simulink model "thermal_project"  (R2021a)
settings: Solver=FixedStepDiscrete  StartTime=0.0  StopTime=10.0  FixedStep=0.1  RelTol=1e-3
libraries: simulink x3
settings Model: Creator=vayne  LastModifiedBy=vayne
settings OptimizationCC: DefaultParameterBehavior=Inlined  EnhancedBackFolding=on  PassReuseOutputArgsAs=Individual arguments  ZeroExternalMemoryAtStartup=off  ZeroInternalMemoryAtStartup=off  OptimizeBlockOrder=speed  DifferentSizesBufferReuse=on  OptimizationCustomize=off  EfficientTunableParamExpr=on
settings DebuggingCC: ParameterTunabilityLossMsg=error
settings HardwareCC: ProdBitPerPointer=32  ProdBitPerSizeT=32  ProdBitPerPtrDiffT=32  ProdLargestAtomicInteger=Long  ProdLargestAtomicFloat=Double  ProdWordSize=32  ProdHWDeviceType=ARM Compatible->ARM Cortex-M
settings SFSimCC: MATLABDynamicMemAlloc=off
settings RTWCC: Description=Create Visual C/C++ Solution File for Embedded Coder  SystemTargetFile=ert.tlc  GenCodeOnly=on  TemplateMakefile=ert_default_tmf  Toolchain=MinGW64 | gmake (64-bit Windows)
settings CodeAppCC: ForceParamTrailComments=on  IgnoreCustomStorageClasses=off  OperatorAnnotations=on  SimulinkDataObjDesc=on  SFDataObjDesc=on  InsertBlockDesc=on
settings ERTTargetCC: TargetLangStandard=C99 (ISO)  GenerateSampleERTMain=on  InlinedParameterPlacement=NonHierarchical  ERTCustomFileTemplate=example_file_process.tlc

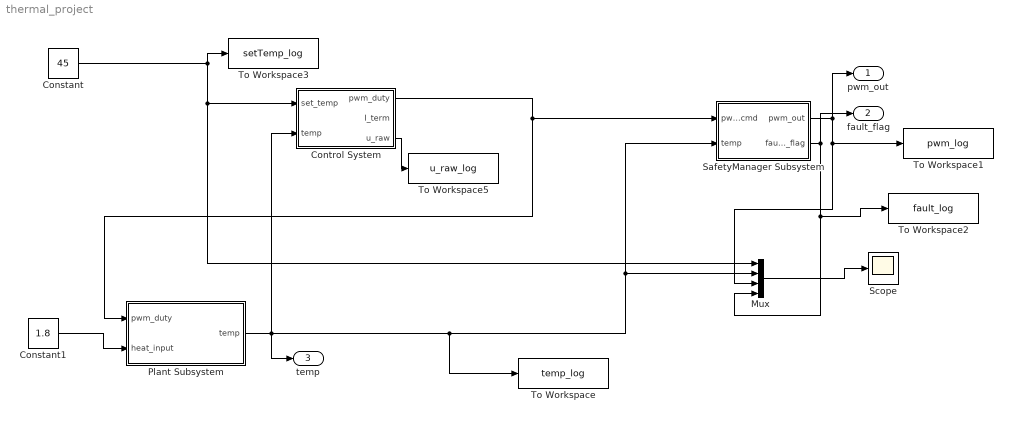
== system thermal_project ==
  Constant : Constant  Value=45
  Constant1 : Constant  Value=1.8
  Control System : Subsystem
  Mux : Mux
  Plant Subsystem : Subsystem
  SafetyManager Subsystem : Subsystem
  Scope : Scope
  To Workspace : ToWorkspace  VariableName=temp_log  SaveFormat=Structure With Time  SampleTime=-1
  To Workspace1 : ToWorkspace  VariableName=pwm_log  SaveFormat=Structure With Time  SampleTime=-1
  To Workspace2 : ToWorkspace  VariableName=fault_log  SaveFormat=Structure With Time  SampleTime=-1
  To Workspace3 : ToWorkspace  VariableName=setTemp_log  SaveFormat=Structure With Time  SampleTime=-1
  To Workspace5 : ToWorkspace  VariableName=u_raw_log  SaveFormat=Structure With Time  SampleTime=-1
  pwm_out : Outport
  fault_flag : Outport  Port=2
  temp : Outport  Port=3
  wires:
  Constant/1 -> Mux/1, Control System/1(set_temp), To Workspace3/1
  Control System/3(u_raw) -> To Workspace5/1
  SafetyManager Subsystem/2(fault_flag) -> To Workspace2/1, Mux/4, fault_flag/1
  Plant Subsystem/1(temp) -> temp/1, Control System/2(temp), To Workspace/1, Mux/2, SafetyManager Subsystem/2(temp)
  Mux/1 -> Scope/1
  SafetyManager Subsystem/1(pwm_out) -> To Workspace1/1, Mux/3, pwm_out/1
  Control System/1(pwm_duty) -> SafetyManager Subsystem/1(pwm_cmd), Plant Subsystem/1(pwm_duty)
  Constant1/1 -> Plant Subsystem/2(heat_input)

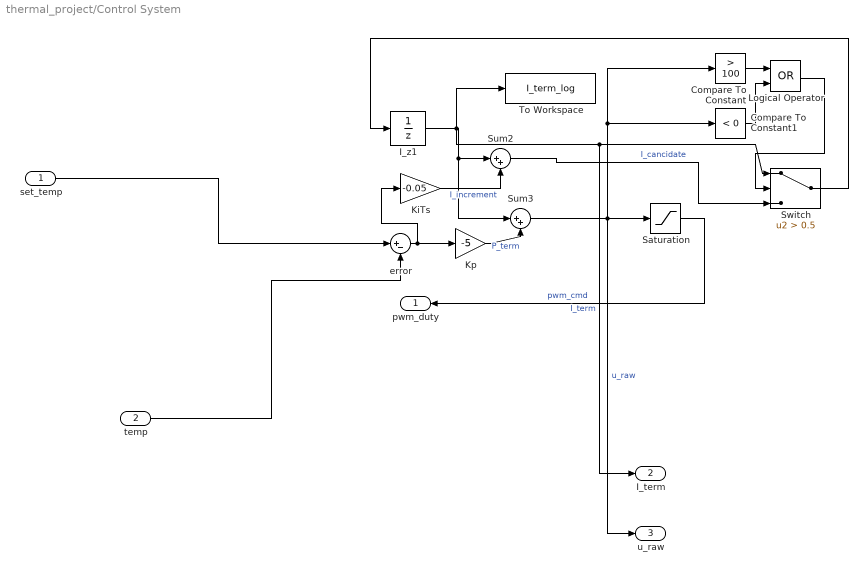
== system thermal_project/Control System ==
  set_temp : Inport
  temp : Inport  Port=2
  Compare To Constant : simulink/Logic and Bit Operations/Compare To Constant  relop=>  const=100  OutDataTypeStr=boolean
  Compare To Constant1 : simulink/Logic and Bit Operations/Compare To Constant  relop=<  const=0  OutDataTypeStr=boolean
  I_z1 : UnitDelay  SampleTime=-1  HasFrameUpgradeWarning=on
  KiTs : Gain  Gain=-0.05
  Kp : Gain  Gain=-5
  Logical Operator : Logic  Operator=OR  AllPortsSameDT=off  OutDataTypeStr=boolean
  Saturation : Saturate  UpperLimit=100  LowerLimit=0
  Sum2 : Sum  Inputs=|++
  Sum3 : Sum  Inputs=|++
  Switch : Switch  Criteria=u2 > Threshold  Threshold=0.5
  To Workspace : ToWorkspace  VariableName=I_term_log  SaveFormat=Structure With Time  SampleTime=-1
  error : Sum  Inputs=|+-
  pwm_duty : Outport
  I_term : Outport  Port=2
  u_raw : Outport  Port=3
  wires:
  error/1 -> KiTs/1, Kp/1
  Sum3/1 -> u_raw/1, Compare To Constant1/1, Compare To Constant/1, Saturation/1  "u_raw"
  set_temp/1 -> error/1
  I_z1/1 -> To Workspace/1, I_term/1, Switch/1, Sum3/1, Sum2/1  "I_term"
  temp/1 -> error/2
  Kp/1 -> Sum3/2  "P_term"
  Sum2/1 -> Switch/3  "I_cancidate"
  KiTs/1 -> Sum2/2  "I_increment"
  Compare To Constant/1 -> Logical Operator/1
  Switch/1 -> I_z1/1
  Logical Operator/1 -> Switch/2
  Compare To Constant1/1 -> Logical Operator/2
  Saturation/1 -> pwm_duty/1  "pwm_cmd"

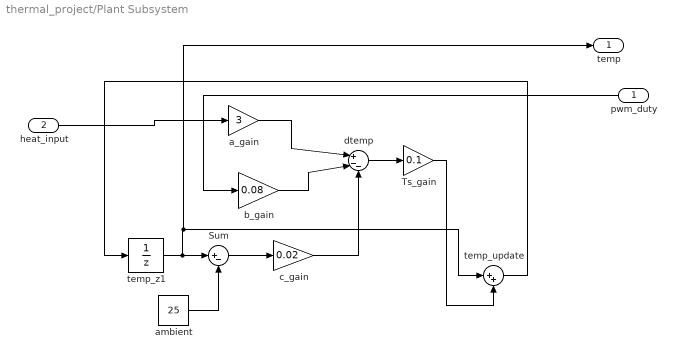
== system thermal_project/Plant Subsystem ==
  pwm_duty : Inport
  heat_input : Inport  Port=2
  Sum : Sum  Inputs=|+-
  Ts_gain : Gain  Gain=0.1
  a_gain : Gain  Gain=3
  ambient : Constant  Value=25
  b_gain : Gain  Gain=0.08
  c_gain : Gain  Gain=0.02
  dtemp : Sum  Inputs=|+--
  temp_update : Sum  Inputs=|++
  temp_z1 : UnitDelay  InitialCondition=25  SampleTime=-1  HasFrameUpgradeWarning=on
  temp : Outport
  wires:
  c_gain/1 -> dtemp/3
  temp_z1/1 -> temp/1, temp_update/1, Sum/1
  a_gain/1 -> dtemp/1
  ambient/1 -> Sum/2
  temp_update/1 -> temp_z1/1
  b_gain/1 -> dtemp/2
  Sum/1 -> c_gain/1
  dtemp/1 -> Ts_gain/1
  Ts_gain/1 -> temp_update/2
  pwm_duty/1 -> b_gain/1
  heat_input/1 -> a_gain/1

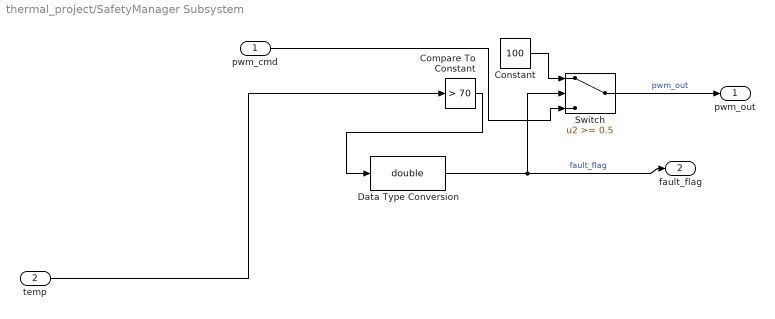
== system thermal_project/SafetyManager Subsystem ==
  pwm_cmd : Inport
  temp : Inport  Port=2
  Compare To Constant : simulink/Logic and Bit Operations/Compare To Constant  relop=>  const=70  OutDataTypeStr=boolean
  Constant : Constant  Value=100
  Data Type Conversion : DataTypeConversion  OutDataTypeStr=double
  Switch : Switch  Threshold=0.5
  pwm_out : Outport
  fault_flag : Outport  Port=2
  wires:
  Switch/1 -> pwm_out/1  "pwm_out"
  Constant/1 -> Switch/1
  pwm_cmd/1 -> Switch/3
  temp/1 -> Compare To Constant/1
  Compare To Constant/1 -> Data Type Conversion/1
  Data Type Conversion/1 -> fault_flag/1, Switch/2  "fault_flag"
